simulink model "Robot_control_pb2"  (R2017b)
settings: Solver=ode45  StartTime=0.0  StopTime=10  RelTol=1e-3
libraries: mblibv1 x4, vrlib x1
settings Model: Creator=zigg  LastModifiedBy=alinvoicu26
settings DataIOCC: SaveFormat=StructureWithTime
settings OptimizationCC: LifeSpan=inf
settings DebuggingCC: FcnCallInpInsideContextMsg=warning  SFExecutionAtInitializationDiag=none
settings HardwareCC: ProdBitPerSizeT=32  ProdBitPerPtrDiffT=32  ProdWordSize=32  ProdHWDeviceType=Specified
settings CodeAppCC: StateflowObjectComments=on

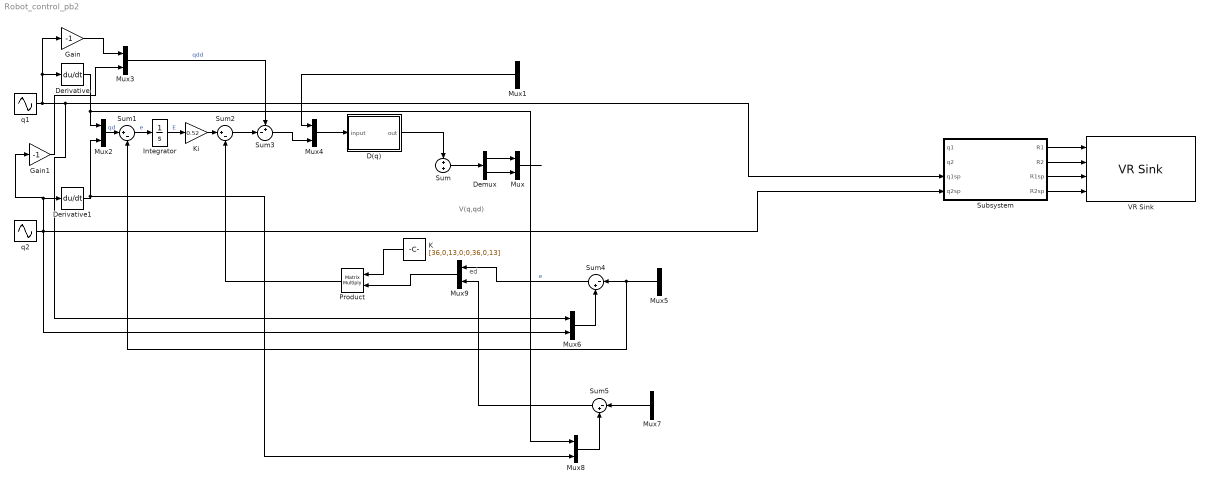
== system Robot_control_pb2 ==
  note: ed
  note: V(q,qd)
  D(q) : MATLAB Function  TreatAsAtomicUnit=on
  Demux : Demux  Outputs=2
  Derivative : Derivative  CoefficientInTFapproximation=100
  Derivative1 : Derivative  CoefficientInTFapproximation=100
  Gain : Gain  Gain=-1
  Gain1 : Gain  Gain=-1
  Integrator : Integrator
  K : Constant  Value=[36,0,13,0;0,36,0,13]
  Ki : Gain  Gain=0.52
  Mux{,1..9} (10 alike) : Mux  Inputs=2
  Product : Product  Multiplication=Matrix(*)
  Subsystem : Subsystem
  Sum : Sum
  Sum1 : Sum  Inputs=|+-
  Sum2 : Sum  Inputs=|+-
  Sum3 : Sum  Inputs=+-|
  Sum4 : Sum  Inputs=|-+
  Sum5 : Sum  Inputs=|-+
  VR Sink : vrlib/VR Sink  InstantiateOnLoad=on  SampleTime=0.1  ViewEnable=on  RemoteChange=off  RemoteView=off  FieldsWritten=Joint1.rotation.4.1.1.double#Joint2.rotation.4.1.1.double#Joint1_SP.rotation.4.1.1.double#Joint2_SP.rotation.4.1.1.double  WorldFileName=my_robot.wrl  AutoView=off  VideoDimensions=[]  AllowVariableSize=off  FigureProperties="{'Position', 'Name', 'Viewpoint', 'CameraBound', 'CameraDirection', 'CameraPosition', 'CameraUpVector', 'ZoomFactor', 'Antialiasing', 'Headlight', 'Lighting', 'NavPanel', 'Sound', 'StatusBar', 'Stereo3D', 'Stereo3DCameraOffset', 'Stereo3DHIT', 'ToolBar', 'Textures', 'Transparency', 'Triad', 'Wireframe', 'NavZones', 'NavMode', 'NavSpeed', 'CaptureFileFormat', 'CaptureFileName', 'Record2DCompressMethod', 'Record2DCompressQuality', 'Record2D', 'Record2DFileName', 'Record2DFPS'; [5.0000000000000000e+00   9.2000000000000000e+01   5.7600000000000000e+02   3.5000000000000000e+02], '', '', 'on', [-2.5899389915367987e-01  -8.7567618684447912e-01  -4.0757008721775917e-01], [8.2878047729177560e+00   2.8021637979023332e+01   1.3042242790968293e+01], [-1.8926568489859164e-01   4.5979838357795461e-01  -8.6761970181581849e-01], [1.0000000000000000e+00], 'on', 'on', 'on', 'halfbar', 'on', 'on', 'off', [1.0000000149011612e-01], [0.0000000000000000e+00], 'on', 'on', 'on', 'none', 'off', 'off', 'examine', 'normal', 'tif', '%f_anim_%n.tif', 'auto', [7.5000000000000000e+01], 'off', '%f_anim_%n.avi', 'auto'}"
      settings: SourceProductBaseCode=VR
  q1 : Sin  Frequency=0.75  SampleTime=0
  q2 : Sin  Frequency=0.5  SampleTime=0
  wires:
  Subsystem/1(R1) -> VR Sink/1
  Subsystem/2(R2) -> VR Sink/2
  Subsystem/3(R1sp) -> VR Sink/3
  Subsystem/4(R2sp) -> VR Sink/4
  ? -> Mux5/1, Subsystem/1(q1), Mux1/1
  ? -> Mux1/2, Mux5/2, Subsystem/2(q2)
  q2/1 -> Mux6/2, Gain1/1, Derivative1/1, Subsystem/4(q2sp)
  Mux/1 -> ?
  ? -> Sum/2
  q1/1 -> Mux6/1, Subsystem/3(q1sp), Gain/1, Derivative/1
  Derivative1/1 -> Mux8/2, Mux2/2
  Derivative/1 -> Mux8/1, Mux2/1
  Mux2/1 -> Sum1/1  "qd"
  Sum1/1 -> Integrator/1  "e"
  Integrator/1 -> Ki/1  "E"
  Ki/1 -> Sum2/1
  Sum2/1 -> Sum3/2
  Gain1/1 -> Mux3/2
  Gain/1 -> Mux3/1
  Mux3/1 -> Sum3/1  "qdd"
  Mux4/1 -> D(q)/1(input)
  Mux1/1 -> Mux4/1
  Sum3/1 -> Mux4/2
  D(q)/1(out) -> Sum/1
  Sum/1 -> Demux/1
  Demux/1 -> Mux/1
  Demux/2 -> Mux/2
  Mux6/1 -> Sum4/2
  Mux8/1 -> Sum5/2
  Mux7/1 -> Sum5/1
  ? -> Mux7/1
  ? -> Mux7/2
  Sum4/1 -> Mux9/1  "e"
  Sum5/1 -> Mux9/2
  Product/1 -> Sum2/2
  Mux5/1 -> Sum1/2, Sum4/1
  Mux9/1 -> Product/2
  K/1 -> Product/1

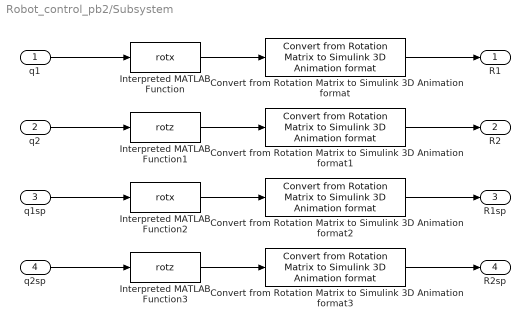
== system Robot_control_pb2/Subsystem ==
  q1 : Inport
  q2 : Inport  Port=2
  q1sp : Inport  Port=3
  q2sp : Inport  Port=4
  Convert from Rotation Matrix to Simulink 3D Animation format{,1..3} (4 alike) : mblibv1/Utilities/Convert from Rotation Matrix to Simulink 3D Animation format
      settings: SourceProductName=Simscape Multibody  SourceProductBaseCode=MS
  Interpreted MATLAB Function : MATLABFcn  MATLABFcn=rotx
  Interpreted MATLAB Function1 : MATLABFcn  MATLABFcn=rotz
  Interpreted MATLAB Function2 : MATLABFcn  MATLABFcn=rotx
  Interpreted MATLAB Function3 : MATLABFcn  MATLABFcn=rotz
  R1 : Outport
  R2 : Outport  Port=2
  R1sp : Outport  Port=3
  R2sp : Outport  Port=4
  wires:
  Convert from Rotation Matrix to Simulink 3D Animation format/1 -> R1/1
  Interpreted MATLAB Function/1 -> Convert from Rotation Matrix to Simulink 3D Animation format/1
  Interpreted MATLAB Function1/1 -> Convert from Rotation Matrix to Simulink 3D Animation format1/1
  Interpreted MATLAB Function2/1 -> Convert from Rotation Matrix to Simulink 3D Animation format2/1
  Interpreted MATLAB Function3/1 -> Convert from Rotation Matrix to Simulink 3D Animation format3/1
  q1/1 -> Interpreted MATLAB Function/1
  q2/1 -> Interpreted MATLAB Function1/1
  q1sp/1 -> Interpreted MATLAB Function2/1
  q2sp/1 -> Interpreted MATLAB Function3/1
  Convert from Rotation Matrix to Simulink 3D Animation format1/1 -> R2/1
  Convert from Rotation Matrix to Simulink 3D Animation format2/1 -> R1sp/1
  Convert from Rotation Matrix to Simulink 3D Animation format3/1 -> R2sp/1

== matlab function Robot_control_pb2/D(q) ==
  data: input input; out output
function out = fcn(input)

    q1 = input(1);
    q2 = input(2);
    A = input(3:4);
    
    out = [0.003515*cos(q2) + 0.000925*cos(q2)^2 + 0.026254, 0;
         0, 0.023625]*A;

end
